simulink model "Grid_modelling_Thermal_V7_ALfix_sheddable_ramped"  (R2025b)
settings: Solver=ode45  StopTime=5000  MaxStep=0.01
libraries: simulink x20, slpidlib x10
(part 3 of 3)

== system Grid_modelling_Thermal_V7_ALfix_sheddable_ramped/source_bus_model_F/Bus_Bar_Thermal_Model ==
  i_src_k : Inport
  Add Constant : Bias  Bias=1  SaturateOnIntegerOverflow=off
  Add1 : Sum
  Constant2 : Constant  Value=25
  Cth_bus : Gain  Gain=1 / 2000
  Integrator1 : Integrator  InitialCondition=25
  Product1 : Product
  Product2 : Product
  R_bus_nom : Constant  Value=0.5e-3
  R_contact : Constant  Value=50e-6
  Rth_bus : Gain  Gain=1/0.6
  Square : Math  Operator=square
  Subtract1 : Sum  Inputs=+-
  Subtract2 : Sum  Inputs=+-
  alpha_copper : Gain  Gain=0.00403
  no_of_contacts : Gain  Gain=10
  T_bus : Outport
  wires:
  Constant2/1 -> Subtract1/2
  Add Constant/1 -> Product2/1
  Product2/1 -> Add1/1
  Cth_bus/1 -> Integrator1/1
  Integrator1/1 -> T_bus/1, Subtract1/1  "T_bus"
  Subtract2/1 -> Cth_bus/1
  alpha_copper/1 -> Add Constant/1
  Subtract1/1 -> alpha_copper/1, Rth_bus/1
  Square/1 -> Product1/1
  Rth_bus/1 -> Subtract2/2
  R_contact/1 -> no_of_contacts/1
  Add1/1 -> Product1/2
  no_of_contacts/1 -> Add1/2
  Product1/1 -> Subtract2/1
  R_bus_nom/1 -> Product2/2
  i_src_k/1 -> Square/1

== system Grid_modelling_Thermal_V7_ALfix_sheddable_ramped/source_bus_model_G/Bus_Bar_Thermal_Model ==
  i_src_k : Inport
  Add Constant : Bias  Bias=1  SaturateOnIntegerOverflow=off
  Add1 : Sum
  Constant2 : Constant  Value=25
  Cth_bus : Gain  Gain=1 / 2000
  Integrator1 : Integrator  InitialCondition=25
  Product1 : Product
  Product2 : Product
  R_bus_nom : Constant  Value=0.5e-3
  R_contact : Constant  Value=50e-6
  Rth_bus : Gain  Gain=1/0.6
  Square : Math  Operator=square
  Subtract1 : Sum  Inputs=+-
  Subtract2 : Sum  Inputs=+-
  alpha_copper : Gain  Gain=0.00403
  no_of_contacts : Gain  Gain=10
  T_bus : Outport
  wires:
  Constant2/1 -> Subtract1/2
  Add Constant/1 -> Product2/1
  Product2/1 -> Add1/1
  Cth_bus/1 -> Integrator1/1
  Integrator1/1 -> T_bus/1, Subtract1/1  "T_bus"
  Subtract2/1 -> Cth_bus/1
  alpha_copper/1 -> Add Constant/1
  Subtract1/1 -> alpha_copper/1, Rth_bus/1
  Square/1 -> Product1/1
  Rth_bus/1 -> Subtract2/2
  R_contact/1 -> no_of_contacts/1
  Add1/1 -> Product1/2
  no_of_contacts/1 -> Add1/2
  Product1/1 -> Subtract2/1
  R_bus_nom/1 -> Product2/2
  i_src_k/1 -> Square/1

== system Grid_modelling_Thermal_V7_ALfix_sheddable_ramped/source_bus_model_H/Bus_Bar_Thermal_Model ==
  i_src_k : Inport
  Add Constant : Bias  Bias=1  SaturateOnIntegerOverflow=off
  Add1 : Sum
  Constant2 : Constant  Value=25
  Cth_bus : Gain  Gain=1 / 2000
  Integrator1 : Integrator  InitialCondition=25
  Product1 : Product
  Product2 : Product
  R_bus_nom : Constant  Value=0.5e-3
  R_contact : Constant  Value=50e-6
  Rth_bus : Gain  Gain=1/0.6
  Square : Math  Operator=square
  Subtract1 : Sum  Inputs=+-
  Subtract2 : Sum  Inputs=+-
  alpha_copper : Gain  Gain=0.00403
  no_of_contacts : Gain  Gain=10
  T_bus : Outport
  wires:
  Constant2/1 -> Subtract1/2
  Add Constant/1 -> Product2/1
  Product2/1 -> Add1/1
  Cth_bus/1 -> Integrator1/1
  Integrator1/1 -> T_bus/1, Subtract1/1  "T_bus"
  Subtract2/1 -> Cth_bus/1
  alpha_copper/1 -> Add Constant/1
  Subtract1/1 -> alpha_copper/1, Rth_bus/1
  Square/1 -> Product1/1
  Rth_bus/1 -> Subtract2/2
  R_contact/1 -> no_of_contacts/1
  Add1/1 -> Product1/2
  no_of_contacts/1 -> Add1/2
  Product1/1 -> Subtract2/1
  R_bus_nom/1 -> Product2/2
  i_src_k/1 -> Square/1

== system Grid_modelling_Thermal_V7_ALfix_sheddable_ramped/source_bus_model_K/Bus_Bar_Thermal_Model ==
  i_src_k : Inport
  Add Constant : Bias  Bias=1  SaturateOnIntegerOverflow=off
  Add1 : Sum
  Constant2 : Constant  Value=25
  Cth_bus : Gain  Gain=1 / 2000
  Integrator1 : Integrator  InitialCondition=25
  Product1 : Product
  Product2 : Product
  R_bus_nom : Constant  Value=0.5e-3
  R_contact : Constant  Value=50e-6
  Rth_bus : Gain  Gain=1/0.6
  Square : Math  Operator=square
  Subtract1 : Sum  Inputs=+-
  Subtract2 : Sum  Inputs=+-
  alpha_copper : Gain  Gain=0.00403
  no_of_contacts : Gain  Gain=10
  T_bus : Outport
  wires:
  Constant2/1 -> Subtract1/2
  Add Constant/1 -> Product2/1
  Product2/1 -> Add1/1
  Cth_bus/1 -> Integrator1/1
  Integrator1/1 -> T_bus/1, Subtract1/1  "T_bus"
  Subtract2/1 -> Cth_bus/1
  alpha_copper/1 -> Add Constant/1
  Subtract1/1 -> alpha_copper/1, Rth_bus/1
  Square/1 -> Product1/1
  Rth_bus/1 -> Subtract2/2
  R_contact/1 -> no_of_contacts/1
  Add1/1 -> Product1/2
  no_of_contacts/1 -> Add1/2
  Product1/1 -> Subtract2/1
  R_bus_nom/1 -> Product2/2
  i_src_k/1 -> Square/1

== system Grid_modelling_Thermal_V7_ALfix_sheddable_ramped/source_bus_model_L/Bus_Bar_Thermal_Model ==
  i_src_k : Inport
  Add Constant : Bias  Bias=1  SaturateOnIntegerOverflow=off
  Add1 : Sum
  Constant2 : Constant  Value=25
  Cth_bus : Gain  Gain=1 / 2000
  Integrator1 : Integrator  InitialCondition=25
  Product1 : Product
  Product2 : Product
  R_bus_nom : Constant  Value=0.5e-3
  R_contact : Constant  Value=50e-6
  Rth_bus : Gain  Gain=1/0.6
  Square : Math  Operator=square
  Subtract1 : Sum  Inputs=+-
  Subtract2 : Sum  Inputs=+-
  alpha_copper : Gain  Gain=0.00403
  no_of_contacts : Gain  Gain=10
  T_bus : Outport
  wires:
  Constant2/1 -> Subtract1/2
  Add Constant/1 -> Product2/1
  Product2/1 -> Add1/1
  Cth_bus/1 -> Integrator1/1
  Integrator1/1 -> T_bus/1, Subtract1/1  "T_bus"
  Subtract2/1 -> Cth_bus/1
  alpha_copper/1 -> Add Constant/1
  Subtract1/1 -> alpha_copper/1, Rth_bus/1
  Square/1 -> Product1/1
  Rth_bus/1 -> Subtract2/2
  R_contact/1 -> no_of_contacts/1
  Add1/1 -> Product1/2
  no_of_contacts/1 -> Add1/2
  Product1/1 -> Subtract2/1
  R_bus_nom/1 -> Product2/2
  i_src_k/1 -> Square/1

== system Grid_modelling_Thermal_V7_ALfix_sheddable_ramped/DAB_Model_AB/thermal_derater/If Action Subsystem ==
  Action Port : ActionPort  ActionPortLabel=if(u1 < 125)
  Constant : Constant
  Out1 : Outport
  wires:
  Constant/1 -> Out1/1

== system Grid_modelling_Thermal_V7_ALfix_sheddable_ramped/DAB_Model_AB/thermal_derater/If Action Subsystem1 ==
  Tj : Inport
  Action Port : ActionPort  ActionPortLabel=elseif(u1 > 125 & u1 < 175)
  Divide : Product  Inputs=*/
  Subtract : Sum  Inputs=+-
  Subtract1 : Sum  Inputs=+-
  Tderate : Constant  Value=125
  Tmax : Constant  Value=175
  Out1 : Outport
  wires:
  Divide/1 -> Out1/1
  Tj/1 -> Subtract/2
  Tmax/1 -> Subtract1/1, Subtract/1
  Tderate/1 -> Subtract1/2
  Subtract/1 -> Divide/1
  Subtract1/1 -> Divide/2

== system Grid_modelling_Thermal_V7_ALfix_sheddable_ramped/DAB_Model_AB/thermal_derater/If Action Subsystem2 ==
  Action Port : ActionPort  ActionPortLabel=elseif( u1 > 175)
  Constant : Constant
  Out1 : Outport
  wires:
  Constant/1 -> Out1/1

== system Grid_modelling_Thermal_V7_ALfix_sheddable_ramped/DAB_Model_AL/thermal_derater/If Action Subsystem ==
  Action Port : ActionPort  ActionPortLabel=if(u1 < 125)
  Constant : Constant
  Out1 : Outport
  wires:
  Constant/1 -> Out1/1

== system Grid_modelling_Thermal_V7_ALfix_sheddable_ramped/DAB_Model_AL/thermal_derater/If Action Subsystem1 ==
  Tj : Inport
  Action Port : ActionPort  ActionPortLabel=elseif(u1 > 125 & u1 < 175)
  Divide : Product  Inputs=*/
  Subtract : Sum  Inputs=+-
  Subtract1 : Sum  Inputs=+-
  Tderate : Constant  Value=125
  Tmax : Constant  Value=175
  Out1 : Outport
  wires:
  Divide/1 -> Out1/1
  Tj/1 -> Subtract/2
  Tmax/1 -> Subtract1/1, Subtract/1
  Tderate/1 -> Subtract1/2
  Subtract/1 -> Divide/1
  Subtract1/1 -> Divide/2

== system Grid_modelling_Thermal_V7_ALfix_sheddable_ramped/DAB_Model_AL/thermal_derater/If Action Subsystem2 ==
  Action Port : ActionPort  ActionPortLabel=elseif( u1 > 175)
  Constant : Constant
  Out1 : Outport
  wires:
  Constant/1 -> Out1/1

== system Grid_modelling_Thermal_V7_ALfix_sheddable_ramped/DAB_Model_BC/thermal_derater/If Action Subsystem ==
  Action Port : ActionPort  ActionPortLabel=if(u1 < 125)
  Constant : Constant
  Out1 : Outport
  wires:
  Constant/1 -> Out1/1

== system Grid_modelling_Thermal_V7_ALfix_sheddable_ramped/DAB_Model_BC/thermal_derater/If Action Subsystem1 ==
  Tj : Inport
  Action Port : ActionPort  ActionPortLabel=elseif(u1 > 125 & u1 < 175)
  Divide : Product  Inputs=*/
  Subtract : Sum  Inputs=+-
  Subtract1 : Sum  Inputs=+-
  Tderate : Constant  Value=125
  Tmax : Constant  Value=175
  Out1 : Outport
  wires:
  Divide/1 -> Out1/1
  Tj/1 -> Subtract/2
  Tmax/1 -> Subtract1/1, Subtract/1
  Tderate/1 -> Subtract1/2
  Subtract/1 -> Divide/1
  Subtract1/1 -> Divide/2

== system Grid_modelling_Thermal_V7_ALfix_sheddable_ramped/DAB_Model_BC/thermal_derater/If Action Subsystem2 ==
  Action Port : ActionPort  ActionPortLabel=elseif( u1 > 175)
  Constant : Constant
  Out1 : Outport
  wires:
  Constant/1 -> Out1/1

== system Grid_modelling_Thermal_V7_ALfix_sheddable_ramped/DAB_Model_CD/thermal_derater/If Action Subsystem ==
  Action Port : ActionPort  ActionPortLabel=if(u1 < 125)
  Constant : Constant
  Out1 : Outport
  wires:
  Constant/1 -> Out1/1

== system Grid_modelling_Thermal_V7_ALfix_sheddable_ramped/DAB_Model_CD/thermal_derater/If Action Subsystem1 ==
  Tj : Inport
  Action Port : ActionPort  ActionPortLabel=elseif(u1 > 125 & u1 < 175)
  Divide : Product  Inputs=*/
  Subtract : Sum  Inputs=+-
  Subtract1 : Sum  Inputs=+-
  Tderate : Constant  Value=125
  Tmax : Constant  Value=175
  Out1 : Outport
  wires:
  Divide/1 -> Out1/1
  Tj/1 -> Subtract/2
  Tmax/1 -> Subtract1/1, Subtract/1
  Tderate/1 -> Subtract1/2
  Subtract/1 -> Divide/1
  Subtract1/1 -> Divide/2

== system Grid_modelling_Thermal_V7_ALfix_sheddable_ramped/DAB_Model_CD/thermal_derater/If Action Subsystem2 ==
  Action Port : ActionPort  ActionPortLabel=elseif( u1 > 175)
  Constant : Constant
  Out1 : Outport
  wires:
  Constant/1 -> Out1/1

== system Grid_modelling_Thermal_V7_ALfix_sheddable_ramped/DAB_Model_DE/thermal_derater/If Action Subsystem ==
  Action Port : ActionPort  ActionPortLabel=if(u1 < 125)
  Constant : Constant
  Out1 : Outport
  wires:
  Constant/1 -> Out1/1

== system Grid_modelling_Thermal_V7_ALfix_sheddable_ramped/DAB_Model_DE/thermal_derater/If Action Subsystem1 ==
  Tj : Inport
  Action Port : ActionPort  ActionPortLabel=elseif(u1 > 125 & u1 < 175)
  Divide : Product  Inputs=*/
  Subtract : Sum  Inputs=+-
  Subtract1 : Sum  Inputs=+-
  Tderate : Constant  Value=125
  Tmax : Constant  Value=175
  Out1 : Outport
  wires:
  Divide/1 -> Out1/1
  Tj/1 -> Subtract/2
  Tmax/1 -> Subtract1/1, Subtract/1
  Tderate/1 -> Subtract1/2
  Subtract/1 -> Divide/1
  Subtract1/1 -> Divide/2

== system Grid_modelling_Thermal_V7_ALfix_sheddable_ramped/DAB_Model_DE/thermal_derater/If Action Subsystem2 ==
  Action Port : ActionPort  ActionPortLabel=elseif( u1 > 175)
  Constant : Constant
  Out1 : Outport
  wires:
  Constant/1 -> Out1/1

== system Grid_modelling_Thermal_V7_ALfix_sheddable_ramped/DAB_Model_EF/thermal_derater/If Action Subsystem ==
  Action Port : ActionPort  ActionPortLabel=if(u1 < 125)
  Constant : Constant
  Out1 : Outport
  wires:
  Constant/1 -> Out1/1

== system Grid_modelling_Thermal_V7_ALfix_sheddable_ramped/DAB_Model_EF/thermal_derater/If Action Subsystem1 ==
  Tj : Inport
  Action Port : ActionPort  ActionPortLabel=elseif(u1 > 125 & u1 < 175)
  Divide : Product  Inputs=*/
  Subtract : Sum  Inputs=+-
  Subtract1 : Sum  Inputs=+-
  Tderate : Constant  Value=125
  Tmax : Constant  Value=175
  Out1 : Outport
  wires:
  Divide/1 -> Out1/1
  Tj/1 -> Subtract/2
  Tmax/1 -> Subtract1/1, Subtract/1
  Tderate/1 -> Subtract1/2
  Subtract/1 -> Divide/1
  Subtract1/1 -> Divide/2

== system Grid_modelling_Thermal_V7_ALfix_sheddable_ramped/DAB_Model_EF/thermal_derater/If Action Subsystem2 ==
  Action Port : ActionPort  ActionPortLabel=elseif( u1 > 175)
  Constant : Constant
  Out1 : Outport
  wires:
  Constant/1 -> Out1/1

== system Grid_modelling_Thermal_V7_ALfix_sheddable_ramped/DAB_Model_FG/thermal_derater/If Action Subsystem ==
  Action Port : ActionPort  ActionPortLabel=if(u1 < 125)
  Constant : Constant
  Out1 : Outport
  wires:
  Constant/1 -> Out1/1

== system Grid_modelling_Thermal_V7_ALfix_sheddable_ramped/DAB_Model_FG/thermal_derater/If Action Subsystem1 ==
  Tj : Inport
  Action Port : ActionPort  ActionPortLabel=elseif(u1 > 125 & u1 < 175)
  Divide : Product  Inputs=*/
  Subtract : Sum  Inputs=+-
  Subtract1 : Sum  Inputs=+-
  Tderate : Constant  Value=125
  Tmax : Constant  Value=175
  Out1 : Outport
  wires:
  Divide/1 -> Out1/1
  Tj/1 -> Subtract/2
  Tmax/1 -> Subtract1/1, Subtract/1
  Tderate/1 -> Subtract1/2
  Subtract/1 -> Divide/1
  Subtract1/1 -> Divide/2

== system Grid_modelling_Thermal_V7_ALfix_sheddable_ramped/DAB_Model_FG/thermal_derater/If Action Subsystem2 ==
  Action Port : ActionPort  ActionPortLabel=elseif( u1 > 175)
  Constant : Constant
  Out1 : Outport
  wires:
  Constant/1 -> Out1/1

== system Grid_modelling_Thermal_V7_ALfix_sheddable_ramped/DAB_Model_GH/thermal_derater/If Action Subsystem ==
  Action Port : ActionPort  ActionPortLabel=if(u1 < 125)
  Constant : Constant
  Out1 : Outport
  wires:
  Constant/1 -> Out1/1

== system Grid_modelling_Thermal_V7_ALfix_sheddable_ramped/DAB_Model_GH/thermal_derater/If Action Subsystem1 ==
  Tj : Inport
  Action Port : ActionPort  ActionPortLabel=elseif(u1 > 125 & u1 < 175)
  Divide : Product  Inputs=*/
  Subtract : Sum  Inputs=+-
  Subtract1 : Sum  Inputs=+-
  Tderate : Constant  Value=125
  Tmax : Constant  Value=175
  Out1 : Outport
  wires:
  Divide/1 -> Out1/1
  Tj/1 -> Subtract/2
  Tmax/1 -> Subtract1/1, Subtract/1
  Tderate/1 -> Subtract1/2
  Subtract/1 -> Divide/1
  Subtract1/1 -> Divide/2

== system Grid_modelling_Thermal_V7_ALfix_sheddable_ramped/DAB_Model_GH/thermal_derater/If Action Subsystem2 ==
  Action Port : ActionPort  ActionPortLabel=elseif( u1 > 175)
  Constant : Constant
  Out1 : Outport
  wires:
  Constant/1 -> Out1/1

== system Grid_modelling_Thermal_V7_ALfix_sheddable_ramped/DAB_Model_HK/thermal_derater/If Action Subsystem ==
  Action Port : ActionPort  ActionPortLabel=if(u1 < 125)
  Constant : Constant
  Out1 : Outport
  wires:
  Constant/1 -> Out1/1

== system Grid_modelling_Thermal_V7_ALfix_sheddable_ramped/DAB_Model_HK/thermal_derater/If Action Subsystem1 ==
  Tj : Inport
  Action Port : ActionPort  ActionPortLabel=elseif(u1 > 125 & u1 < 175)
  Divide : Product  Inputs=*/
  Subtract : Sum  Inputs=+-
  Subtract1 : Sum  Inputs=+-
  Tderate : Constant  Value=125
  Tmax : Constant  Value=175
  Out1 : Outport
  wires:
  Divide/1 -> Out1/1
  Tj/1 -> Subtract/2
  Tmax/1 -> Subtract1/1, Subtract/1
  Tderate/1 -> Subtract1/2
  Subtract/1 -> Divide/1
  Subtract1/1 -> Divide/2

== system Grid_modelling_Thermal_V7_ALfix_sheddable_ramped/DAB_Model_HK/thermal_derater/If Action Subsystem2 ==
  Action Port : ActionPort  ActionPortLabel=elseif( u1 > 175)
  Constant : Constant
  Out1 : Outport
  wires:
  Constant/1 -> Out1/1

== system Grid_modelling_Thermal_V7_ALfix_sheddable_ramped/DAB_Model_KL/thermal_derater/If Action Subsystem ==
  Action Port : ActionPort  ActionPortLabel=if(u1 < 125)
  Constant : Constant
  Out1 : Outport
  wires:
  Constant/1 -> Out1/1

== system Grid_modelling_Thermal_V7_ALfix_sheddable_ramped/DAB_Model_KL/thermal_derater/If Action Subsystem1 ==
  Tj : Inport
  Action Port : ActionPort  ActionPortLabel=elseif(u1 > 125 & u1 < 175)
  Divide : Product  Inputs=*/
  Subtract : Sum  Inputs=+-
  Subtract1 : Sum  Inputs=+-
  Tderate : Constant  Value=125
  Tmax : Constant  Value=175
  Out1 : Outport
  wires:
  Divide/1 -> Out1/1
  Tj/1 -> Subtract/2
  Tmax/1 -> Subtract1/1, Subtract/1
  Tderate/1 -> Subtract1/2
  Subtract/1 -> Divide/1
  Subtract1/1 -> Divide/2

== system Grid_modelling_Thermal_V7_ALfix_sheddable_ramped/DAB_Model_KL/thermal_derater/If Action Subsystem2 ==
  Action Port : ActionPort  ActionPortLabel=elseif( u1 > 175)
  Constant : Constant
  Out1 : Outport
  wires:
  Constant/1 -> Out1/1
